simulink model "main_copy"  (R2023b)
settings: Solver=ode4  StartTime=0.0  StopTime=20  FixedStep=0.0001  RelTol=1e-3  AbsTol=1e-3  EnableMultiTasking=on
undefined symbols (not defined in the file or in its folder): X, Y, Z
libraries: sm_lib x84, nesl_utility x13, simulink_extras x3, ArmLibrary x2, gripper_v2_bottom x2, gripper_v2_top x2, lower_link_v2 x1, WorkSpaceLibrarry x1
settings Model: Creator=thiwa  LastModifiedBy=thiwa
settings SolverCC: AutoScaleAbsTol=off  AlgebraicLoopSolver=TrustRegion  MaxZcPerStep=1
settings DataIOCC: LimitDataPoints=on  MaxDataPoints=10000
settings OptimizationCC: ReuseModelBlockBuffer=off  LifeSpan=inf
settings DebuggingCC: UnconnectedInputMsg=warning  UnconnectedOutputMsg=warning  UnconnectedLineMsg=warning  AllowSymbolicDim=off  SubsystemReferenceDiagnosticForUnitTest=warning  SFUnexpectedBacktrackingDiag=warning  SFNoUnconditionalDefaultTransitionDiag=warning  SFExecutionAtInitializationDiag=none  ArithmeticOperatorsInVariantConditions=warning
settings ModelReferenceCC: EnableRefExpFcnMdlSchedulingChecks=on
settings SFSimCC: SimUseLocalCustomCode=off  CustomCodeUndefinedFunction=UseInterfaceOnly
settings RTWCC: RTWUseLocalCustomCode=off  DLArmComputeVersion=19.05
settings CodeAppCC: StateflowObjectComments=on
settings GRTTargetCC: TargetLangStandard=C89/C90 (ANSI)
settings ConfigComp: CovMetricSettings=dw  CovSaveCumulativeToWorkspaceVar=on  CovSaveSingleToWorkspaceVar=on  CovExternalEMLEnable=off  CovSFcnEnable=off
settings SimscapeCC: SimscapeLogType=all  SimscapeLogSimulationStatistics=on  SimscapeLogDataHistory=10000

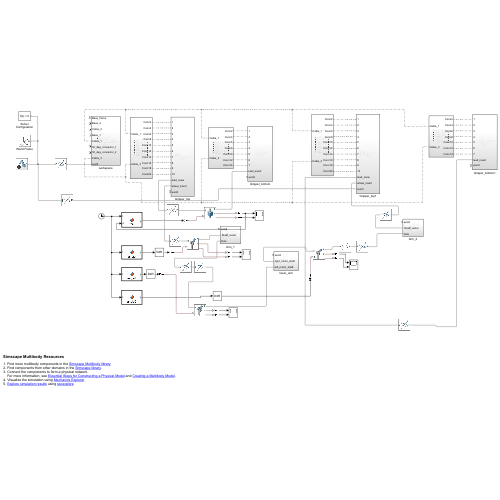
[thumbnail: Simulink's stored preview of the top-level diagram]
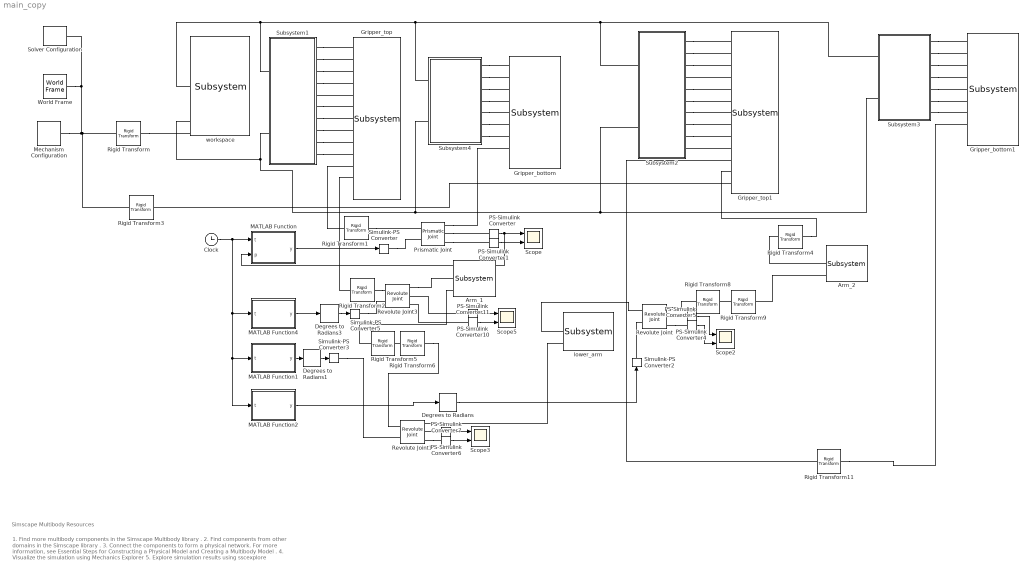
== system main_copy ==
  note: 1. Find more multibody components in the Simscape Multibody library .
      | 2. Find components from other domains in the Simscape library .
      | 3. Connect the components to form a physical network.
      | For more information, see Essential Steps for Constructing a Physical Model and Creating a Multibody Model .
      | 4. Visualize the simulation using Mechanics Explorer
      | 5. Explore simulation results using sscexplore
  note: Simscape Multibody Resources
  Arm_1 : ArmLibrary/Subsystem  SystemSampleTime=-1  VariantActivationTime=update diagram  AllowFlexibleInterface=on  Latency=0  AutoFrameSizeCalculation=off
  Arm_2 : ArmLibrary/Subsystem  SystemSampleTime=-1  VariantActivationTime=update diagram  AllowFlexibleInterface=on  Latency=0  AutoFrameSizeCalculation=off
  Clock : Clock
  Degrees to Radians : simulink_extras/Transformations/Degrees to Radians
  Degrees to Radians1 : simulink_extras/Transformations/Degrees to Radians
  Degrees to Radians3 : simulink_extras/Transformations/Degrees to Radians
  Gripper_bottom : gripper_v2_bottom/Subsystem  SystemSampleTime=-1  VariantActivationTime=update diagram  AllowFlexibleInterface=on  Latency=0  AutoFrameSizeCalculation=off
  Gripper_bottom1 : gripper_v2_bottom/Subsystem  SystemSampleTime=-1  VariantActivationTime=update diagram  AllowFlexibleInterface=on  Latency=0  AutoFrameSizeCalculation=off
  Gripper_top : gripper_v2_top/Subsystem  SystemSampleTime=-1  VariantActivationTime=update diagram  AllowFlexibleInterface=on  Latency=0  AutoFrameSizeCalculation=off
  Gripper_top1 : gripper_v2_top/Subsystem  SystemSampleTime=-1  VariantActivationTime=update diagram  AllowFlexibleInterface=on  Latency=0  AutoFrameSizeCalculation=off
  MATLAB Function : MATLAB Function  TreatAsAtomicUnit=on
  MATLAB Function1 : MATLAB Function  TreatAsAtomicUnit=on
  MATLAB Function2 : MATLAB Function  TreatAsAtomicUnit=on
  MATLAB Function4 : MATLAB Function  TreatAsAtomicUnit=on
  Mechanism Configuration : sm_lib/Utilities/Mechanism Configuration  UniformGravity=Constant  GravityVector=[0 0 -9.80665]  GravityVectorUnits=m/s^2  LinearizationDelta=0.001  JointModeTransitionNonlinearIterations=3
  PS-Simulink Converter{,1,4,6..7,10..11} (7 alike) : nesl_utility/PS-Simulink Converter  PhysicalDomain=network_engine_domain  SubClassName=ps_output  LeftPortType=input  RightPortType=output  PseudoPeriodic=off  Frequencies=[]  VectorFormat=inherit  Unit=inherit  AffineConversion=off
  PS-Simulink Converter5 : nesl_utility/PS-Simulink Converter  PhysicalDomain=network_engine_domain  SubClassName=ps_output  LeftPortType=input  RightPortType=output  PseudoPeriodic=off  Frequencies=[]  VectorFormat=inherit  Unit=N*m  AffineConversion=off
  Prismatic Joint : sm_lib/Joints/Prismatic Joint  JointMode=Normal  SenseConstraintForce=off  SenseConstraintForceX=off  SenseConstraintForceY=off  SenseConstraintForceZ=off  SenseConstraintTorque=off  SenseConstraintTorqueX=off  SenseConstraintTorqueY=off  SenseConstraintTorqueZ=off  SenseTotalForce=off  SenseTotalForceX=off  SenseTotalForceY=off  SenseTotalForceZ=off  SenseTotalTorque=off  SenseTotalTorqueX=off  SenseTotalTorqueY=off  SenseTotalTorqueZ=off  CompositeWrenchDir=FollowerOnBase  CompositeWrenchFrame=BaseFrame  EquilibriumPosition=0  EquilibriumPositionUnits=m  SpringStiffness=0  SpringStiffnessUnits=N/m  DampingCoefficient=10  DampingCoefficientUnits=N/(m/s)  TorqueActuationMode=InputTorque  MotionActuationMode=ComputedMotion  SensePosition=on  SenseVelocity=off  SenseAcceleration=off  SenseTorqueForce=on  SenseLowerLimitTorqueForce=off  SenseUpperLimitTorqueForce=off  LowerLimitSpecify=off  LowerLimitBound=-1  LowerLimitBoundUnits=m  LowerLimitStiffness=1e6  LowerLimitStiffnessUnits=N/m  LowerLimitDamping=1e3  LowerLimitDampingUnits=N/(m/s)  LowerLimitTransitionRegionWidth=1e-4  LowerLimitTransitionRegionWidthUnits=m  UpperLimitSpecify=off  UpperLimitBound=1  UpperLimitBoundUnits=m  UpperLimitStiffness=1e6  UpperLimitStiffnessUnits=N/m  UpperLimitDamping=1e3  UpperLimitDampingUnits=N/(m/s)  UpperLimitTransitionRegionWidth=1e-4  UpperLimitTransitionRegionWidthUnits=m  PositionTargetSpecify=on  PositionTargetPriority=High  PositionTargetValue=-50  PositionTargetValueUnits=mm  VelocityTargetSpecify=off  VelocityTargetPriority=High  VelocityTargetValue=0  VelocityTargetValueUnits=m/s
  Revolute Joint : sm_lib/Joints/Revolute Joint  JointMode=Normal  SenseConstraintForce=off  SenseConstraintForceX=off  SenseConstraintForceY=off  SenseConstraintForceZ=off  SenseConstraintTorque=off  SenseConstraintTorqueX=off  SenseConstraintTorqueY=off  SenseConstraintTorqueZ=off  SenseTotalForce=off  SenseTotalForceX=off  SenseTotalForceY=off  SenseTotalForceZ=off  SenseTotalTorque=off  SenseTotalTorqueX=off  SenseTotalTorqueY=off  SenseTotalTorqueZ=off  CompositeWrenchDir=FollowerOnBase  CompositeWrenchFrame=BaseFrame  EquilibriumPosition=0  EquilibriumPositionUnits=deg  SpringStiffness=0  SpringStiffnessUnits=N*m/deg  DampingCoefficient=1  DampingCoefficientUnits=N*m/(deg/s)  TorqueActuationMode=ComputedTorque  MotionActuationMode=InputMotion  SensePosition=on  SenseVelocity=off  SenseAcceleration=off  SenseTorqueForce=on  SenseLowerLimitTorqueForce=off  SenseUpperLimitTorqueForce=off  LowerLimitSpecify=off  LowerLimitBound=-90  LowerLimitBoundUnits=deg  LowerLimitStiffness=1e4  LowerLimitStiffnessUnits=N*m/deg  LowerLimitDamping=10  LowerLimitDampingUnits=N*m/(deg/s)  LowerLimitTransitionRegionWidth=0.1  LowerLimitTransitionRegionWidthUnits=deg  UpperLimitSpecify=off  UpperLimitBound=90  UpperLimitBoundUnits=deg  UpperLimitStiffness=1e4  UpperLimitStiffnessUnits=N*m/deg  UpperLimitDamping=10  UpperLimitDampingUnits=N*m/(deg/s)  UpperLimitTransitionRegionWidth=0.1  UpperLimitTransitionRegionWidthUnits=deg  PositionTargetSpecify=on  PositionTargetPriority=High  PositionTargetValue=0  PositionTargetValueUnits=deg  VelocityTargetSpecify=off  VelocityTargetPriority=High  VelocityTargetValue=0  VelocityTargetValueUnits=deg/s
  Revolute Joint1 : sm_lib/Joints/Revolute Joint  JointMode=Normal  SenseConstraintForce=off  SenseConstraintForceX=off  SenseConstraintForceY=off  SenseConstraintForceZ=off  SenseConstraintTorque=off  SenseConstraintTorqueX=off  SenseConstraintTorqueY=off  SenseConstraintTorqueZ=off  SenseTotalForce=off  SenseTotalForceX=off  SenseTotalForceY=off  SenseTotalForceZ=off  SenseTotalTorque=off  SenseTotalTorqueX=off  SenseTotalTorqueY=off  SenseTotalTorqueZ=off  CompositeWrenchDir=FollowerOnBase  CompositeWrenchFrame=BaseFrame  EquilibriumPosition=0  EquilibriumPositionUnits=deg  SpringStiffness=0  SpringStiffnessUnits=N*m/deg  DampingCoefficient=1  DampingCoefficientUnits=N*m/(deg/s)  TorqueActuationMode=ComputedTorque  MotionActuationMode=InputMotion  SensePosition=on  SenseVelocity=off  SenseAcceleration=off  SenseTorqueForce=on  SenseLowerLimitTorqueForce=off  SenseUpperLimitTorqueForce=off  LowerLimitSpecify=off  LowerLimitBound=-90  LowerLimitBoundUnits=deg  LowerLimitStiffness=1e4  LowerLimitStiffnessUnits=N*m/deg  LowerLimitDamping=10  LowerLimitDampingUnits=N*m/(deg/s)  LowerLimitTransitionRegionWidth=0.1  LowerLimitTransitionRegionWidthUnits=deg  UpperLimitSpecify=off  UpperLimitBound=90  UpperLimitBoundUnits=deg  UpperLimitStiffness=1e4  UpperLimitStiffnessUnits=N*m/deg  UpperLimitDamping=10  UpperLimitDampingUnits=N*m/(deg/s)  UpperLimitTransitionRegionWidth=0.1  UpperLimitTransitionRegionWidthUnits=deg  PositionTargetSpecify=on  PositionTargetPriority=High  PositionTargetValue=-90  PositionTargetValueUnits=deg  VelocityTargetSpecify=off  VelocityTargetPriority=High  VelocityTargetValue=0  VelocityTargetValueUnits=deg/s
  Revolute Joint3 : sm_lib/Joints/Revolute Joint  JointMode=Normal  SenseConstraintForce=off  SenseConstraintForceX=off  SenseConstraintForceY=off  SenseConstraintForceZ=off  SenseConstraintTorque=off  SenseConstraintTorqueX=off  SenseConstraintTorqueY=off  SenseConstraintTorqueZ=off  SenseTotalForce=off  SenseTotalForceX=off  SenseTotalForceY=off  SenseTotalForceZ=off  SenseTotalTorque=off  SenseTotalTorqueX=off  SenseTotalTorqueY=off  SenseTotalTorqueZ=off  CompositeWrenchDir=FollowerOnBase  CompositeWrenchFrame=BaseFrame  EquilibriumPosition=0  EquilibriumPositionUnits=deg  SpringStiffness=0  SpringStiffnessUnits=N*m/deg  DampingCoefficient=1  DampingCoefficientUnits=N*m/(deg/s)  TorqueActuationMode=ComputedTorque  MotionActuationMode=InputMotion  SensePosition=on  SenseVelocity=off  SenseAcceleration=off  SenseTorqueForce=on  SenseLowerLimitTorqueForce=off  SenseUpperLimitTorqueForce=off  LowerLimitSpecify=off  LowerLimitBound=-90  LowerLimitBoundUnits=deg  LowerLimitStiffness=1e4  LowerLimitStiffnessUnits=N*m/deg  LowerLimitDamping=10  LowerLimitDampingUnits=N*m/(deg/s)  LowerLimitTransitionRegionWidth=0.1  LowerLimitTransitionRegionWidthUnits=deg  UpperLimitSpecify=off  UpperLimitBound=90  UpperLimitBoundUnits=deg  UpperLimitStiffness=1e4  UpperLimitStiffnessUnits=N*m/deg  UpperLimitDamping=10  UpperLimitDampingUnits=N*m/(deg/s)  UpperLimitTransitionRegionWidth=0.1  UpperLimitTransitionRegionWidthUnits=deg  PositionTargetSpecify=on  PositionTargetPriority=High  PositionTargetValue=-90-25.5  PositionTargetValueUnits=deg  VelocityTargetSpecify=off  VelocityTargetPriority=High  VelocityTargetValue=0  VelocityTargetValueUnits=deg/s
  Rigid Transform : sm_lib/Frames and Transforms/Rigid Transform  TranslationMethod=None  TranslationStandardOffset=0  TranslationStandardOffsetUnits=m  TranslationStandardAxis=+Z  TranslationCartesianOffset=[0 0 0]  TranslationCartesianOffsetUnits=m  TranslationROffset=0  TranslationROffsetUnits=m  TranslationZOffset=0  TranslationZOffsetUnits=m  TranslationThetaOffset=0  TranslationThetaOffsetUnits=deg  RotationMethod=StandardAxis  RotationAngleUnits=deg  RotationStandardAxis=+Y  RotationAngle=180  RotationArbitraryAxis=[0 0 1]  FollAlignAxisA=+X  BaseAlignAxisA=+Y  FollAlignAxisB=+Y  BaseAlignAxisB=+Z  RotationSequenceAxes=FollowerAxes  RotationSequence=XYX  RotationSequenceAngles=[0 0 0]  RotationSequenceAnglesUnits=deg  RotationMatrix=[1 0 0; 0 1 0; 0 0 1]  Quaternion=[1 0 0 0]
  Rigid Transform1 : sm_lib/Frames and Transforms/Rigid Transform  TranslationMethod=None  TranslationStandardOffset=0  TranslationStandardOffsetUnits=m  TranslationStandardAxis=+Z  TranslationCartesianOffset=[0 0 0]  TranslationCartesianOffsetUnits=m  TranslationROffset=0  TranslationROffsetUnits=m  TranslationZOffset=0  TranslationZOffsetUnits=m  TranslationThetaOffset=0  TranslationThetaOffsetUnits=deg  RotationMethod=StandardAxis  RotationAngleUnits=deg  RotationStandardAxis=+Y  RotationAngle=180  RotationArbitraryAxis=[0 0 1]  FollAlignAxisA=+X  BaseAlignAxisA=+Y  FollAlignAxisB=+Y  BaseAlignAxisB=+Z  RotationSequenceAxes=FollowerAxes  RotationSequence=XYX  RotationSequenceAngles=[0 0 0]  RotationSequenceAnglesUnits=deg  RotationMatrix=[1 0 0; 0 1 0; 0 0 1]  Quaternion=[1 0 0 0]
  Rigid Transform11 : sm_lib/Frames and Transforms/Rigid Transform  TranslationMethod=StandardAxis  TranslationStandardOffset=50  TranslationStandardOffsetUnits=mm  TranslationStandardAxis=+Z  TranslationCartesianOffset=[0 0 0]  TranslationCartesianOffsetUnits=m  TranslationROffset=0  TranslationROffsetUnits=m  TranslationZOffset=0  TranslationZOffsetUnits=m  TranslationThetaOffset=0  TranslationThetaOffsetUnits=deg  RotationMethod=StandardAxis  RotationAngleUnits=deg  RotationStandardAxis=+Y  RotationAngle=180  RotationArbitraryAxis=[0 0 1]  FollAlignAxisA=+X  BaseAlignAxisA=+Y  FollAlignAxisB=+Y  BaseAlignAxisB=+Z  RotationSequenceAxes=FollowerAxes  RotationSequence=XYX  RotationSequenceAngles=[0 0 0]  RotationSequenceAnglesUnits=deg  RotationMatrix=[1 0 0; 0 1 0; 0 0 1]  Quaternion=[1 0 0 0]
  Rigid Transform2 : sm_lib/Frames and Transforms/Rigid Transform  TranslationMethod=StandardAxis  TranslationStandardOffset=12  TranslationStandardOffsetUnits=mm  TranslationStandardAxis=-Z  TranslationCartesianOffset=[0 0 0]  TranslationCartesianOffsetUnits=m  TranslationROffset=0  TranslationROffsetUnits=m  TranslationZOffset=0  TranslationZOffsetUnits=m  TranslationThetaOffset=0  TranslationThetaOffsetUnits=deg  RotationMethod=None  RotationAngleUnits=deg  RotationStandardAxis=+Z  RotationAngle=0.0  RotationArbitraryAxis=[0 0 1]  FollAlignAxisA=+X  BaseAlignAxisA=+Y  FollAlignAxisB=+Y  BaseAlignAxisB=+Z  RotationSequenceAxes=FollowerAxes  RotationSequence=XYX  RotationSequenceAngles=[0 0 0]  RotationSequenceAnglesUnits=deg  RotationMatrix=[1 0 0; 0 1 0; 0 0 1]  Quaternion=[1 0 0 0]
  Rigid Transform3 : sm_lib/Frames and Transforms/Rigid Transform  TranslationMethod=None  TranslationStandardOffset=0  TranslationStandardOffsetUnits=m  TranslationStandardAxis=+Z  TranslationCartesianOffset=[0 0 0]  TranslationCartesianOffsetUnits=m  TranslationROffset=0  TranslationROffsetUnits=m  TranslationZOffset=0  TranslationZOffsetUnits=m  TranslationThetaOffset=0  TranslationThetaOffsetUnits=deg  RotationMethod=StandardAxis  RotationAngleUnits=deg  RotationStandardAxis=+Y  RotationAngle=180  RotationArbitraryAxis=[0 0 1]  FollAlignAxisA=+X  BaseAlignAxisA=+Y  FollAlignAxisB=+Y  BaseAlignAxisB=+Z  RotationSequenceAxes=FollowerAxes  RotationSequence=XYX  RotationSequenceAngles=[0 0 0]  RotationSequenceAnglesUnits=deg  RotationMatrix=[1 0 0; 0 1 0; 0 0 1]  Quaternion=[1 0 0 0]
  Rigid Transform4 : sm_lib/Frames and Transforms/Rigid Transform  TranslationMethod=None  TranslationStandardOffset=0  TranslationStandardOffsetUnits=m  TranslationStandardAxis=+Z  TranslationCartesianOffset=[0 0 0]  TranslationCartesianOffsetUnits=m  TranslationROffset=0  TranslationROffsetUnits=m  TranslationZOffset=0  TranslationZOffsetUnits=m  TranslationThetaOffset=0  TranslationThetaOffsetUnits=deg  RotationMethod=StandardAxis  RotationAngleUnits=deg  RotationStandardAxis=+Z  RotationAngle=25.5+90  RotationArbitraryAxis=[0 0 1]  FollAlignAxisA=+X  BaseAlignAxisA=+Y  FollAlignAxisB=+Y  BaseAlignAxisB=+Z  RotationSequenceAxes=FollowerAxes  RotationSequence=XYX  RotationSequenceAngles=[0 0 0]  RotationSequenceAnglesUnits=deg  RotationMatrix=[1 0 0; 0 1 0; 0 0 1]  Quaternion=[1 0 0 0]
  Rigid Transform5 : sm_lib/Frames and Transforms/Rigid Transform  TranslationMethod=None  TranslationStandardOffset=0  TranslationStandardOffsetUnits=m  TranslationStandardAxis=+Z  TranslationCartesianOffset=[0 0 0]  TranslationCartesianOffsetUnits=m  TranslationROffset=0  TranslationROffsetUnits=m  TranslationZOffset=0  TranslationZOffsetUnits=m  TranslationThetaOffset=0  TranslationThetaOffsetUnits=deg  RotationMethod=StandardAxis  RotationAngleUnits=deg  RotationStandardAxis=+Y  RotationAngle=90  RotationArbitraryAxis=[0 0 1]  FollAlignAxisA=+X  BaseAlignAxisA=+Y  FollAlignAxisB=+Y  BaseAlignAxisB=+Z  RotationSequenceAxes=FollowerAxes  RotationSequence=XYX  RotationSequenceAngles=[0 0 0]  RotationSequenceAnglesUnits=deg  RotationMatrix=[1 0 0; 0 1 0; 0 0 1]  Quaternion=[1 0 0 0]
  Rigid Transform6 : sm_lib/Frames and Transforms/Rigid Transform  TranslationMethod=None  TranslationStandardOffset=0  TranslationStandardOffsetUnits=m  TranslationStandardAxis=+Z  TranslationCartesianOffset=[0 0 0]  TranslationCartesianOffsetUnits=m  TranslationROffset=0  TranslationROffsetUnits=m  TranslationZOffset=0  TranslationZOffsetUnits=m  TranslationThetaOffset=0  TranslationThetaOffsetUnits=deg  RotationMethod=StandardAxis  RotationAngleUnits=deg  RotationStandardAxis=+X  RotationAngle=180  RotationArbitraryAxis=[0 0 1]  FollAlignAxisA=+X  BaseAlignAxisA=+Y  FollAlignAxisB=+Y  BaseAlignAxisB=+Z  RotationSequenceAxes=FollowerAxes  RotationSequence=XYX  RotationSequenceAngles=[0 0 0]  RotationSequenceAnglesUnits=deg  RotationMatrix=[1 0 0; 0 1 0; 0 0 1]  Quaternion=[1 0 0 0]
  Rigid Transform8 : sm_lib/Frames and Transforms/Rigid Transform  TranslationMethod=None  TranslationStandardOffset=0  TranslationStandardOffsetUnits=m  TranslationStandardAxis=+Z  TranslationCartesianOffset=[0 0 0]  TranslationCartesianOffsetUnits=m  TranslationROffset=0  TranslationROffsetUnits=m  TranslationZOffset=0  TranslationZOffsetUnits=m  TranslationThetaOffset=0  TranslationThetaOffsetUnits=deg  RotationMethod=StandardAxis  RotationAngleUnits=deg  RotationStandardAxis=+Y  RotationAngle=90  RotationArbitraryAxis=[0 0 1]  FollAlignAxisA=+X  BaseAlignAxisA=+Y  FollAlignAxisB=+Y  BaseAlignAxisB=+Z  RotationSequenceAxes=FollowerAxes  RotationSequence=XYX  RotationSequenceAngles=[0 0 0]  RotationSequenceAnglesUnits=deg  RotationMatrix=[1 0 0; 0 1 0; 0 0 1]  Quaternion=[1 0 0 0]
  Rigid Transform9 : sm_lib/Frames and Transforms/Rigid Transform  TranslationMethod=None  TranslationStandardOffset=0  TranslationStandardOffsetUnits=m  TranslationStandardAxis=+Z  TranslationCartesianOffset=[0 0 0]  TranslationCartesianOffsetUnits=m  TranslationROffset=0  TranslationROffsetUnits=m  TranslationZOffset=0  TranslationZOffsetUnits=m  TranslationThetaOffset=0  TranslationThetaOffsetUnits=deg  RotationMethod=StandardAxis  RotationAngleUnits=deg  RotationStandardAxis=+X  RotationAngle=90  RotationArbitraryAxis=[0 0 1]  FollAlignAxisA=+X  BaseAlignAxisA=+Y  FollAlignAxisB=+Y  BaseAlignAxisB=+Z  RotationSequenceAxes=FollowerAxes  RotationSequence=XYX  RotationSequenceAngles=[0 0 0]  RotationSequenceAnglesUnits=deg  RotationMatrix=[1 0 0; 0 1 0; 0 0 1]  Quaternion=[1 0 0 0]
  Scope{,2..3,5} (4 alike) : Scope  NumInputPorts=2
  Simulink-PS Converter : nesl_utility/Simulink-PS Converter  PhysicalDomain=network_engine_domain  SubClassName=ps_input  LeftPortType=input  RightPortType=output  PseudoPeriodic=off  Frequencies=[]  NoiseDistribution=none  NoiseParameters=[]  Unit=1  AffineConversion=off  FilteringAndDerivatives=provide  SimscapeFilterOrder=1  InputFilterTimeConstant=0.001  UdotUserProvided=0
  Simulink-PS Converter2 : nesl_utility/Simulink-PS Converter  PhysicalDomain=network_engine_domain  SubClassName=ps_input  LeftPortType=input  RightPortType=output  PseudoPeriodic=off  Frequencies=[]  NoiseDistribution=none  NoiseParameters=[]  Unit=1  AffineConversion=off  FilteringAndDerivatives=filter  SimscapeFilterOrder=2  InputFilterTimeConstant=0.001  UdotUserProvided=0
  Simulink-PS Converter3 : nesl_utility/Simulink-PS Converter  PhysicalDomain=network_engine_domain  SubClassName=ps_input  LeftPortType=input  RightPortType=output  PseudoPeriodic=off  Frequencies=[]  NoiseDistribution=none  NoiseParameters=[]  Unit=1  AffineConversion=off  FilteringAndDerivatives=filter  SimscapeFilterOrder=2  InputFilterTimeConstant=0.001  UdotUserProvided=0
  Simulink-PS Converter5 : nesl_utility/Simulink-PS Converter  PhysicalDomain=network_engine_domain  SubClassName=ps_input  LeftPortType=input  RightPortType=output  PseudoPeriodic=off  Frequencies=[]  NoiseDistribution=none  NoiseParameters=[]  Unit=1  AffineConversion=off  FilteringAndDerivatives=filter  SimscapeFilterOrder=2  InputFilterTimeConstant=0.001  UdotUserProvided=0
  Solver Configuration : nesl_utility/Solver Configuration  PhysicalDomain=network_engine_domain  SubClassName=solver  LeftPortType=input  RightPortType=generic  Tones=[]  Harmonics=[]  SimulateNoise=off  Profile=off  UseLocalSampling=off  EnableSwitchedLinearOptims=on  FrequencyDomain=off  UseCCode=off  RelTol=0.001  AbsTol=1e-06  MinStep=1e-09  ToWorkspace=off  RevertToSquareIcSolve=off  NumHomotopyIterations=100  PhasorMode=off  PhasorModeNumHarmonics=1  ConsistencySolver=NEWTON_XTOL_AFTER_FTOL  IndexReductionMethod=DerivativeReplacement  DoDC=off  ResidualTolerance=1e-09  ConsistencyTolSource=GLOBAL  ConsistencyAbsTol=0.001  ConsistencyRelTol=0.001  ConsistencyTolFactor=0.001  UseLocalSolver=off  LocalSolverChoice=NE_BACKWARD_EULER_ADVANCER  ResolveIndetEquations=on  FunctionEvalNumThread=1  LocalSolverSampleTime=0.001  DoFixedCost=off  MaxNonlinIter=3  MaxModeIter=2  ComputeImpulses=off  ImpulseIterations=2  LinearAlgebra=Sparse  LinearAlgebraNumThread=0  EquationFormulation=NE_TIME_EF  DelaysMemoryBudget=1024  AutomaticFiltering=on  FilteringTimeConstant=0.001  PartitionStorageMethod=AS_NEEDED  PartitionMemoryBudget=1024  PartitionMethod=FAST  MultibodyUseLocalSolver=off  MultibodyLocalSolverChoice=ODE1  MultibodyLocalSolverSampleTime=0.001
  Subsystem1 : Subsystem
  Subsystem2 : Subsystem
  Subsystem3 : Subsystem
  Subsystem4 : Subsystem
  World Frame : sm_lib/Frames and Transforms/World Frame
  lower_arm : lower_link_v2/Subsystem  SystemSampleTime=-1  VariantActivationTime=update diagram  AllowFlexibleInterface=on  Latency=0  AutoFrameSizeCalculation=off
  workspace : WorkSpaceLibrarry/Subsystem  SystemSampleTime=-1  VariantActivationTime=update diagram  AllowFlexibleInterface=on  Latency=0  AutoFrameSizeCalculation=off
      link override Cable_3_RIGID/Solid: ExtGeomFileName=C:\Thiwanka\Assignments\Cable_Inspection_Robot\Design\Simscapetest_3\Workspace_Frame\Cable_100_long_sldprt.STEP
  wires:
  PS-Simulink Converter1/1 -> Scope/2
  PS-Simulink Converter/1 -> MATLAB Function/2(p), Scope/1
  MATLAB Function/1(y) -> Simulink-PS Converter/1
  Clock/1 -> MATLAB Function/1(t), MATLAB Function4/1(t), MATLAB Function1/1(t), MATLAB Function2/1(t)
  PS-Simulink Converter7/1 -> Scope3/2
  PS-Simulink Converter6/1 -> Scope3/1
  Degrees to Radians1/1 -> Simulink-PS Converter3/1
  MATLAB Function1/1(y) -> Degrees to Radians1/1
  PS-Simulink Converter10/1 -> Scope5/1
  PS-Simulink Converter11/1 -> Scope5/2
  Degrees to Radians3/1 -> Simulink-PS Converter5/1
  MATLAB Function4/1(y) -> Degrees to Radians3/1
  MATLAB Function2/1(y) -> Degrees to Radians/1
  Degrees to Radians/1 -> Simulink-PS Converter2/1
  PS-Simulink Converter4/1 -> Scope2/1
  PS-Simulink Converter5/1 -> Scope2/2
  connections:
  Rigid Transform/RConn1 -- workspace/LConn9
  Prismatic Joint/RConn1 -- Gripper_bottom/LConn8
  Rigid Transform2/LConn1 -- Gripper_top/LConn12
  Rigid Transform6/LConn1 -- Rigid Transform5/RConn1
  Rigid Transform9/LConn1 -- Rigid Transform8/RConn1
  Rigid Transform11/LConn1 -- Gripper_top1/LConn11
  Rigid Transform1/RConn1 -- Prismatic Joint/LConn1
  Prismatic Joint/RConn2 -- PS-Simulink Converter/LConn1
  Prismatic Joint/RConn3 -- PS-Simulink Converter1/LConn1
  Simulink-PS Converter/RConn1 -- Prismatic Joint/LConn2
  Rigid Transform11/RConn1 -- Gripper_bottom1/LConn8
  World Frame/RConn1 -- Rigid Transform3/LConn1 -- Rigid Transform/LConn1 -- Mechanism Configuration/RConn1 -- Solver Configuration/RConn1
  lower_arm/LConn2 -- Revolute Joint/LConn1
  Revolute Joint/RConn1 -- Rigid Transform8/LConn1
  Revolute Joint1/RConn2 -- PS-Simulink Converter6/LConn1
  Revolute Joint1/RConn3 -- PS-Simulink Converter7/LConn1
  Simulink-PS Converter3/RConn1 -- Revolute Joint1/LConn2
  Rigid Transform5/LConn1 -- Arm_1/LConn3
  Rigid Transform6/RConn1 -- Revolute Joint1/LConn1
  Revolute Joint1/RConn1 -- lower_arm/LConn3
  Subsystem4/RConn1 -- Gripper_bottom/LConn1
  Subsystem4/RConn2 -- Gripper_bottom/LConn2
  Subsystem4/RConn3 -- Gripper_bottom/LConn3
  Subsystem4/RConn4 -- Gripper_bottom/LConn4
  Subsystem4/RConn5 -- Gripper_bottom/LConn5
  Subsystem4/RConn6 -- Gripper_bottom/LConn6
  Subsystem4/RConn7 -- Gripper_bottom/LConn7
  Subsystem1/RConn10 -- Gripper_top/LConn10
  Subsystem1/RConn9 -- Gripper_top/LConn9
  Subsystem1/RConn8 -- Gripper_top/LConn8
  Subsystem1/RConn7 -- Gripper_top/LConn7
  Subsystem1/RConn6 -- Gripper_top/LConn6
  Gripper_top/LConn5 -- Subsystem1/RConn5
  Subsystem1/RConn4 -- Gripper_top/LConn4
  Subsystem1/RConn3 -- Gripper_top/LConn3
  Subsystem1/RConn2 -- Gripper_top/LConn2
  Subsystem1/RConn1 -- Gripper_top/LConn1
  workspace/LConn5 -- Subsystem3/LConn1 -- Subsystem2/LConn1 -- Subsystem4/LConn1 -- Subsystem1/LConn1
  Subsystem1/LConn2 -- Subsystem2/LConn2 -- Subsystem3/LConn2 -- Subsystem4/LConn2 -- workspace/LConn8
  Subsystem2/RConn1 -- Gripper_top1/LConn1
  Subsystem2/RConn2 -- Gripper_top1/LConn2
  Subsystem2/RConn3 -- Gripper_top1/LConn3
  Gripper_top1/LConn4 -- Subsystem2/RConn4
  Subsystem2/RConn5 -- Gripper_top1/LConn5
  Subsystem2/RConn6 -- Gripper_top1/LConn6
  Subsystem2/RConn7 -- Gripper_top1/LConn7
  Subsystem2/RConn8 -- Gripper_top1/LConn8
  Subsystem2/RConn9 -- Gripper_top1/LConn9
  Gripper_top1/LConn10 -- Subsystem2/RConn10
  Subsystem3/RConn1 -- Gripper_bottom1/LConn1
  Subsystem3/RConn2 -- Gripper_bottom1/LConn2
  Subsystem3/RConn3 -- Gripper_bottom1/LConn3
  Subsystem3/RConn4 -- Gripper_bottom1/LConn4
  Subsystem3/RConn5 -- Gripper_bottom1/LConn5
  Subsystem3/RConn6 -- Gripper_bottom1/LConn6
  Subsystem3/RConn7 -- Gripper_bottom1/LConn7
  Rigid Transform2/RConn1 -- Revolute Joint3/LConn1
  Revolute Joint3/RConn1 -- Arm_1/LConn2
  PS-Simulink Converter10/LConn1 -- Revolute Joint3/RConn2
  PS-Simulink Converter11/LConn1 -- Revolute Joint3/RConn3
  Simulink-PS Converter5/RConn1 -- Revolute Joint3/LConn2
  Arm_2/LConn3 -- Rigid Transform9/RConn1
  Simulink-PS Converter2/RConn1 -- Revolute Joint/LConn2
  Revolute Joint/RConn2 -- PS-Simulink Converter4/LConn1
  Revolute Joint/RConn3 -- PS-Simulink Converter5/LConn1
  Gripper_top/LConn11 -- Rigid Transform1/LConn1
  Gripper_top1/LConn13 -- Rigid Transform3/RConn1
  Arm_2/LConn2 -- Rigid Transform4/LConn1
  Rigid Transform4/RConn1 -- Gripper_top1/LConn12

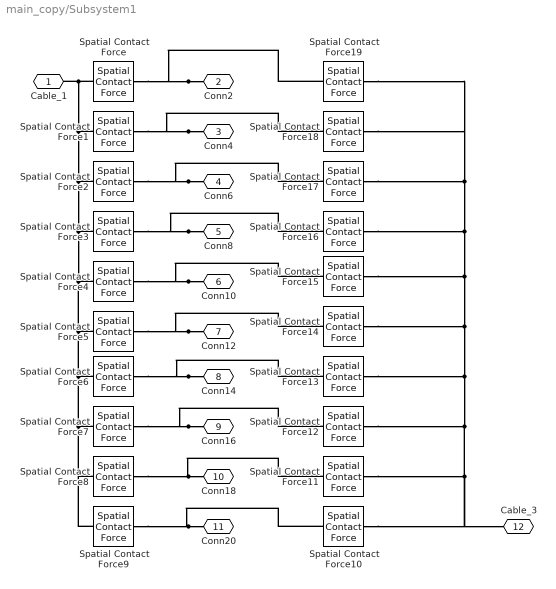
== system main_copy/Subsystem1 ==
  Spatial Contact Force{,1..19} (20 alike) : sm_lib/Forces and Torques/Spatial Contact Force  SenseContactBaseRotation=off  SenseContactBaseTranslation=off  CoefficientOfDynamicFriction=0.3  CoefficientOfStaticFriction=0.5  NormalDamping=1e3  NormalDampingUnits=N/(m/s)  SenseContactSignal=off  NormalStiffness=1e6  NormalStiffnessUnits=N/m  FrictionalCriticalVelocity=1e-3  FrictionalCriticalVelocityUnits=m/s  ZeroCrossDetectContactStartAndEnd=off  SenseContactFollowerRotation=off  SenseContactFollowerTranslation=off  FrictionType=SmoothStickSlip  SenseFrictionalForceMagnitude=off  SenseNormalForceMagnitude=off  NormalForceType=SmoothSpringDamper  SenseNormalVelocity=off  SensePenetrationDepth=off  SenseSeparationDistance=off  SenseTangentialVelocity=off  NormalTransitionRegionWidth=1e-4  NormalTransitionRegionWidthUnits=m
  Cable_1 : PMIOPort  Side=Left
  Conn2 : PMIOPort  Port=2  Side=Right
  Conn4 : PMIOPort  Port=3  Side=Right
  Conn6 : PMIOPort  Port=4  Side=Right
  Conn8 : PMIOPort  Port=5  Side=Right
  Conn10 : PMIOPort  Port=6  Side=Right
  Conn12 : PMIOPort  Port=7  Side=Right
  Conn14 : PMIOPort  Port=8  Side=Right
  Conn16 : PMIOPort  Port=9  Side=Right
  Conn18 : PMIOPort  Port=10  Side=Right
  Conn20 : PMIOPort  Port=11  Side=Right
  Cable_3 : PMIOPort  Port=12  Side=Left
  connections:
  Spatial Contact Force15/LConn1 -- Spatial Contact Force14/LConn1 -- Spatial Contact Force13/LConn1 -- Spatial Contact Force11/LConn1 -- Cable_3/RConn1 -- Spatial Contact Force10/LConn1 -- Spatial Contact Force12/LConn1 -- Spatial Contact Force17/LConn1 -- Spatial Contact Force18/LConn1 -- Spatial Contact Force19/LConn1 -- Spatial Contact Force16/LConn1
  Conn20/RConn1 -- Spatial Contact Force10/RConn1 -- Spatial Contact Force9/RConn1
  Conn16/RConn1 -- Spatial Contact Force12/RConn1 -- Spatial Contact Force7/RConn1
  Conn18/RConn1 -- Spatial Contact Force11/RConn1 -- Spatial Contact Force8/RConn1
  Conn14/RConn1 -- Spatial Contact Force13/RConn1 -- Spatial Contact Force6/RConn1
  Conn8/RConn1 -- Spatial Contact Force16/RConn1 -- Spatial Contact Force3/RConn1
  Conn10/RConn1 -- Spatial Contact Force15/RConn1 -- Spatial Contact Force4/RConn1
  Conn12/RConn1 -- Spatial Contact Force14/RConn1 -- Spatial Contact Force5/RConn1
  Conn6/RConn1 -- Spatial Contact Force17/RConn1 -- Spatial Contact Force2/RConn1
  Cable_1/RConn1 -- Spatial Contact Force1/LConn1 -- Spatial Contact Force2/LConn1 -- Spatial Contact Force3/LConn1 -- Spatial Contact Force4/LConn1 -- Spatial Contact Force5/LConn1 -- Spatial Contact Force6/LConn1 -- Spatial Contact Force7/LConn1 -- Spatial Contact Force8/LConn1 -- Spatial Contact Force9/LConn1 -- Spatial Contact Force/LConn1
  Conn4/RConn1 -- Spatial Contact Force18/RConn1 -- Spatial Contact Force1/RConn1
  Conn2/RConn1 -- Spatial Contact Force19/RConn1 -- Spatial Contact Force/RConn1

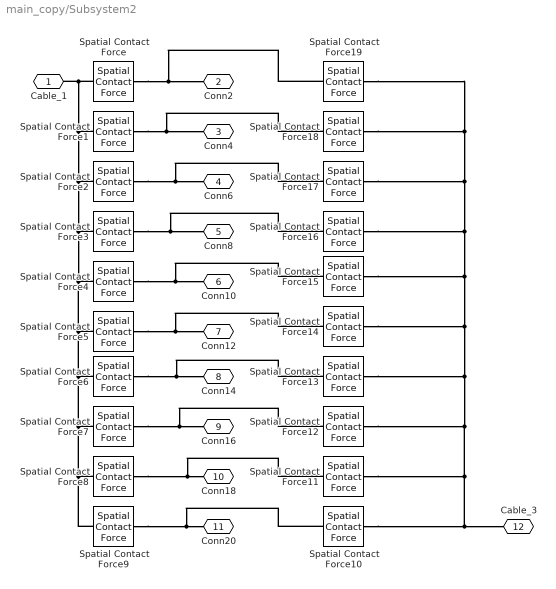
== system main_copy/Subsystem2 ==
  Spatial Contact Force{,1..19} (20 alike) : sm_lib/Forces and Torques/Spatial Contact Force  SenseContactBaseRotation=off  SenseContactBaseTranslation=off  CoefficientOfDynamicFriction=0.3  CoefficientOfStaticFriction=0.5  NormalDamping=1e3  NormalDampingUnits=N/(m/s)  SenseContactSignal=off  NormalStiffness=1e6  NormalStiffnessUnits=N/m  FrictionalCriticalVelocity=1e-3  FrictionalCriticalVelocityUnits=m/s  ZeroCrossDetectContactStartAndEnd=off  SenseContactFollowerRotation=off  SenseContactFollowerTranslation=off  FrictionType=SmoothStickSlip  SenseFrictionalForceMagnitude=off  SenseNormalForceMagnitude=off  NormalForceType=SmoothSpringDamper  SenseNormalVelocity=off  SensePenetrationDepth=off  SenseSeparationDistance=off  SenseTangentialVelocity=off  NormalTransitionRegionWidth=1e-4  NormalTransitionRegionWidthUnits=m
  Cable_1 : PMIOPort  Side=Left
  Conn2 : PMIOPort  Port=2  Side=Right
  Conn4 : PMIOPort  Port=3  Side=Right
  Conn6 : PMIOPort  Port=4  Side=Right
  Conn8 : PMIOPort  Port=5  Side=Right
  Conn10 : PMIOPort  Port=6  Side=Right
  Conn12 : PMIOPort  Port=7  Side=Right
  Conn14 : PMIOPort  Port=8  Side=Right
  Conn16 : PMIOPort  Port=9  Side=Right
  Conn18 : PMIOPort  Port=10  Side=Right
  Conn20 : PMIOPort  Port=11  Side=Right
  Cable_3 : PMIOPort  Port=12  Side=Left
  connections:
  Spatial Contact Force/RConn1 -- Spatial Contact Force19/RConn1 -- Conn2/RConn1
  Spatial Contact Force1/RConn1 -- Spatial Contact Force18/RConn1 -- Conn4/RConn1
  Spatial Contact Force/LConn1 -- Spatial Contact Force9/LConn1 -- Spatial Contact Force8/LConn1 -- Spatial Contact Force7/LConn1 -- Spatial Contact Force6/LConn1 -- Spatial Contact Force5/LConn1 -- Spatial Contact Force4/LConn1 -- Spatial Contact Force3/LConn1 -- Spatial Contact Force2/LConn1 -- Spatial Contact Force1/LConn1 -- Cable_1/RConn1
  Spatial Contact Force2/RConn1 -- Spatial Contact Force17/RConn1 -- Conn6/RConn1
  Spatial Contact Force5/RConn1 -- Spatial Contact Force14/RConn1 -- Conn12/RConn1
  Spatial Contact Force4/RConn1 -- Spatial Contact Force15/RConn1 -- Conn10/RConn1
  Spatial Contact Force3/RConn1 -- Spatial Contact Force16/RConn1 -- Conn8/RConn1
  Spatial Contact Force6/RConn1 -- Spatial Contact Force13/RConn1 -- Conn14/RConn1
  Spatial Contact Force8/RConn1 -- Spatial Contact Force11/RConn1 -- Conn18/RConn1
  Spatial Contact Force7/RConn1 -- Spatial Contact Force12/RConn1 -- Conn16/RConn1
  Spatial Contact Force9/RConn1 -- Spatial Contact Force10/RConn1 -- Conn20/RConn1
  Spatial Contact Force16/LConn1 -- Spatial Contact Force19/LConn1 -- Spatial Contact Force18/LConn1 -- Spatial Contact Force17/LConn1 -- Spatial Contact Force12/LConn1 -- Spatial Contact Force10/LConn1 -- Cable_3/RConn1 -- Spatial Contact Force11/LConn1 -- Spatial Contact Force13/LConn1 -- Spatial Contact Force14/LConn1 -- Spatial Contact Force15/LConn1

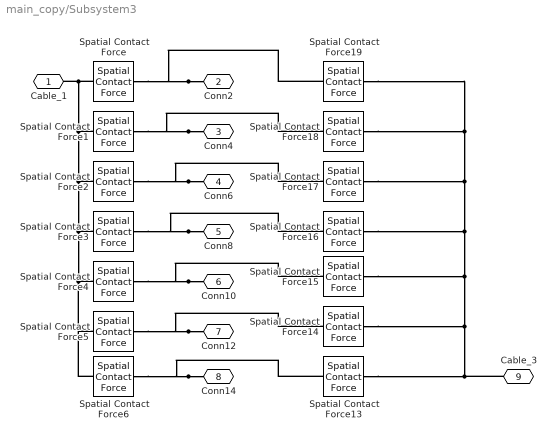
== system main_copy/Subsystem3 ==
  Spatial Contact Force{,1..6,13..19} (14 alike) : sm_lib/Forces and Torques/Spatial Contact Force  SenseContactBaseRotation=off  SenseContactBaseTranslation=off  CoefficientOfDynamicFriction=0.3  CoefficientOfStaticFriction=0.5  NormalDamping=1e3  NormalDampingUnits=N/(m/s)  SenseContactSignal=off  NormalStiffness=1e6  NormalStiffnessUnits=N/m  FrictionalCriticalVelocity=1e-3  FrictionalCriticalVelocityUnits=m/s  ZeroCrossDetectContactStartAndEnd=off  SenseContactFollowerRotation=off  SenseContactFollowerTranslation=off  FrictionType=SmoothStickSlip  SenseFrictionalForceMagnitude=off  SenseNormalForceMagnitude=off  NormalForceType=SmoothSpringDamper  SenseNormalVelocity=off  SensePenetrationDepth=off  SenseSeparationDistance=off  SenseTangentialVelocity=off  NormalTransitionRegionWidth=1e-4  NormalTransitionRegionWidthUnits=m
  Cable_1 : PMIOPort  Side=Left
  Conn2 : PMIOPort  Port=2  Side=Right
  Conn4 : PMIOPort  Port=3  Side=Right
  Conn6 : PMIOPort  Port=4  Side=Right
  Conn8 : PMIOPort  Port=5  Side=Right
  Conn10 : PMIOPort  Port=6  Side=Right
  Conn12 : PMIOPort  Port=7  Side=Right
  Conn14 : PMIOPort  Port=8  Side=Right
  Cable_3 : PMIOPort  Port=9  Side=Left
  connections:
  Conn2/RConn1 -- Spatial Contact Force/RConn1 -- Spatial Contact Force19/RConn1
  Conn4/RConn1 -- Spatial Contact Force1/RConn1 -- Spatial Contact Force18/RConn1
  Spatial Contact Force/LConn1 -- Cable_1/RConn1 -- Spatial Contact Force1/LConn1 -- Spatial Contact Force2/LConn1 -- Spatial Contact Force3/LConn1 -- Spatial Contact Force4/LConn1 -- Spatial Contact Force6/LConn1 -- Spatial Contact Force5/LConn1
  Conn6/RConn1 -- Spatial Contact Force2/RConn1 -- Spatial Contact Force17/RConn1
  Conn12/RConn1 -- Spatial Contact Force5/RConn1 -- Spatial Contact Force14/RConn1
  Conn10/RConn1 -- Spatial Contact Force4/RConn1 -- Spatial Contact Force15/RConn1
  Conn8/RConn1 -- Spatial Contact Force3/RConn1 -- Spatial Contact Force16/RConn1
  Conn14/RConn1 -- Spatial Contact Force6/RConn1 -- Spatial Contact Force13/RConn1
  Spatial Contact Force19/LConn1 -- Spatial Contact Force18/LConn1 -- Spatial Contact Force17/LConn1 -- Spatial Contact Force16/LConn1 -- Spatial Contact Force15/LConn1 -- Spatial Contact Force14/LConn1 -- Cable_3/RConn1 -- Spatial Contact Force13/LConn1

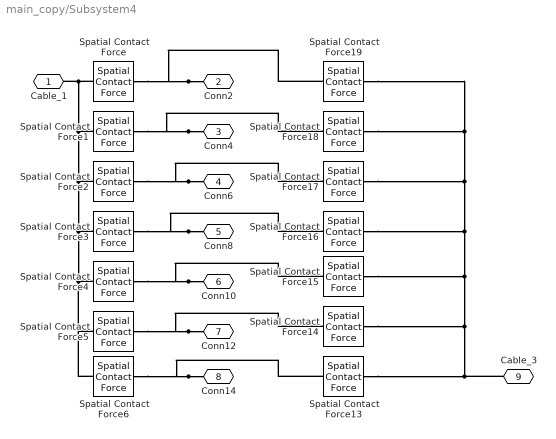
== system main_copy/Subsystem4 ==
  Spatial Contact Force{,1..6,13..19} (14 alike) : sm_lib/Forces and Torques/Spatial Contact Force  SenseContactBaseRotation=off  SenseContactBaseTranslation=off  CoefficientOfDynamicFriction=0.3  CoefficientOfStaticFriction=0.5  NormalDamping=1e3  NormalDampingUnits=N/(m/s)  SenseContactSignal=off  NormalStiffness=1e6  NormalStiffnessUnits=N/m  FrictionalCriticalVelocity=1e-3  FrictionalCriticalVelocityUnits=m/s  ZeroCrossDetectContactStartAndEnd=off  SenseContactFollowerRotation=off  SenseContactFollowerTranslation=off  FrictionType=SmoothStickSlip  SenseFrictionalForceMagnitude=off  SenseNormalForceMagnitude=off  NormalForceType=SmoothSpringDamper  SenseNormalVelocity=off  SensePenetrationDepth=off  SenseSeparationDistance=off  SenseTangentialVelocity=off  NormalTransitionRegionWidth=1e-4  NormalTransitionRegionWidthUnits=m
  Cable_1 : PMIOPort  Side=Left
  Conn2 : PMIOPort  Port=2  Side=Right
  Conn4 : PMIOPort  Port=3  Side=Right
  Conn6 : PMIOPort  Port=4  Side=Right
  Conn8 : PMIOPort  Port=5  Side=Right
  Conn10 : PMIOPort  Port=6  Side=Right
  Conn12 : PMIOPort  Port=7  Side=Right
  Conn14 : PMIOPort  Port=8  Side=Right
  Cable_3 : PMIOPort  Port=9  Side=Left
  connections:
  Conn2/RConn1 -- Spatial Contact Force/RConn1 -- Spatial Contact Force19/RConn1
  Conn4/RConn1 -- Spatial Contact Force1/RConn1 -- Spatial Contact Force18/RConn1
  Spatial Contact Force/LConn1 -- Cable_1/RConn1 -- Spatial Contact Force1/LConn1 -- Spatial Contact Force2/LConn1 -- Spatial Contact Force3/LConn1 -- Spatial Contact Force4/LConn1 -- Spatial Contact Force6/LConn1 -- Spatial Contact Force5/LConn1
  Conn6/RConn1 -- Spatial Contact Force2/RConn1 -- Spatial Contact Force17/RConn1
  Conn12/RConn1 -- Spatial Contact Force5/RConn1 -- Spatial Contact Force14/RConn1
  Conn10/RConn1 -- Spatial Contact Force4/RConn1 -- Spatial Contact Force15/RConn1
  Conn8/RConn1 -- Spatial Contact Force3/RConn1 -- Spatial Contact Force16/RConn1
  Conn14/RConn1 -- Spatial Contact Force6/RConn1 -- Spatial Contact Force13/RConn1
  Spatial Contact Force19/LConn1 -- Spatial Contact Force18/LConn1 -- Spatial Contact Force17/LConn1 -- Spatial Contact Force16/LConn1 -- Spatial Contact Force15/LConn1 -- Spatial Contact Force14/LConn1 -- Cable_3/RConn1 -- Spatial Contact Force13/LConn1

== matlab function main_copy/MATLAB Function1 ==
  data: t input; y output
function y = angle2(t)

    % Each row represents one motion:
    % [t_start, duration, y_start, y_end]

    movements = [
        1.5, 1.0,   -90,   -96;
        3.5, 2.0,  -96,   0;
        11.5, 4.0,  0,  90;
    ];

    % Initial value
    y = movements(1,3);

    % Check each motion
    for i = 1:size(movements,1)

        t_start = movements(i,1);
        duration = movements(i,2);
        y_start = movements(i,3);
        y_end = movements(i,4);

        % Before this movement
        if t <= t_start

            y = y_start;
            return

        % During this movement
        elseif t < (t_start + duration)

            % Normalized time: 0 -> 1
            tau = (t - t_start) / duration;

            % 5th-order smooth trajectory
            s = 6*tau^5 - 15*tau^4 + 10*tau^3;

            y = y_start + (y_end - y_start) * s;
            return

        % After this movement
        else

            y = y_end;

        end
    end
end

== matlab function main_copy/MATLAB Function ==
  data: t input; y output; p input
function y = fcn(t, p) 
    % ===================================================================== 
    % CONTROL PARAMETERS 
    % ===================================================================== 
    F_clamp             = -0;    % Target full clamping force (N) 
     
    % --- Initial Clamping Parameters --- 
    F_approach1         = -1;     % Gentle approach force for first clamp (N) 
    p_stiffness1        = 0.002;    % Penetration depth for full force (m) 
     
    % --- Second Clamping Parameters (Specific to final phase) --- 
    F_approach_clamp2   = -0.001;     % Gentle approach force for second clamp (N) 
    p_stiffness_clamp2  = 0.0015;   % Penetration depth for second clamp (m) 
     
    p_contact           = 0.0;      % Contact position threshold (m) 
     
    p_start             = -0.015;   % Position when clamped (m) 
    p_target            = -15e-3;     % Target release position (m) 
     
    t_release           = 0.5;      % Time to start release (s) 
    move_dur            = 0.8;      % Duration of release movement (s) 
     
    Kp                  = 150;      % Position tracking gain (N/m) 
    Kd_scale            = 0.5;      % Braking scale when overshooting 
     
    t_second_clamp      = 16.5;      % Time to re-engage clamping (s) 
    % ===================================================================== 
    p_start2 = 0.06; 
    p_target2 =0; 
     
    % 1. Initial Clamping Phase 
    if t < t_release 
        if p < p_contact 
            % Gentle approach before contact 
            y = F_approach1; 
        else 
            % Smooth force ramp upon contact based on deflection 
            contact_ratio = min(1.0, (p - p_contact) / p_stiffness1); 
            y = F_approach1 + (F_clamp - F_approach1) * contact_ratio; 
        end 
         
    % 2. S-Curve Release & Dynamic Hold Phase 
    elseif t >= t_release && t < (t_second_clamp-1.5) 
        tau = min(1.0, (t - t_release) / move_dur); 
         
        s_curve = tau^3 * (6 * tau^2 - 15 * tau + 10); 
        p_ref = p_start + (p_target - p_start) * s_curve; 
         
        err = p_ref - p; 
        p_start2=p; 
        if err >= 0 
            y = Kp * err; 
        else 
            y = Kp * err * (1 + Kd_scale * abs(err)); 
        end 
         
        if tau >= 1.0 
            if abs(p_target - p) < 0.003 
                y = y * (abs(p_target - p) / 0.003); 
            end 
        end 
         
    % 3. Second Clamping Phase (t >= t_second_clamp) 
    elseif t > (t_second_clamp-1.5)  && t <t_second_clamp 
        tau = min(1.0, (t - (t_second_clamp-1.5)) / move_dur); 
         
        s_curve = tau^3 * (6 * tau^2 - 15 * tau + 10); 
        p_ref = p_start2 + (p_target2 - p_start2) * s_curve; 
         
        err = p_ref - p; 
         
        if err >= 0 
            y = Kp * err; 
        else 
            y = Kp * err * (1 + Kd_scale * abs(err)); 
        end 
         
        if tau >= 1.0 
            if abs(p_target2 - p) < 0.003 
                y = y * (abs(p_target2 - p) / 0.003); 
            end 
        end 
    else 
        y = -500; 
    end 
end

== matlab function main_copy/MATLAB Function2 ==
  data: t input; y output

function y = angle2(t)

    % Each row represents one motion:
    % [t_start, duration, y_start, y_end]

    movements = [
      
        1.5, 1.0,   0,   -6;
        5.5, 4.0,   -6,   186;

    ];

    % Initial position
    y = movements(1,3);

    % Check each movement
    for i = 1:size(movements,1)

        t_start = movements(i,1);
        duration = movements(i,2);
        y_start = movements(i,3);
        y_end = movements(i,4);

        if t <= t_start

            % Before movement starts
            y = y_start;
            return

        elseif t < (t_start + duration)

            % During movement
            tau = (t - t_start) / duration;

            % 5th-order smooth trajectory
            s = 6*tau^5 - 15*tau^4 + 10*tau^3;

            y = y_start + (y_end - y_start) * s;
            return

        else

            % Movement completed
            y = y_end;

        end
    end
end

== matlab function main_copy/MATLAB Function4 ==
  data: t input; y output
function y = angle(t)

    % Each row represents one movement:
    % [t_start, duration, y_start, y_end]

    movements = [
        3.0, 0.5,   -90-25.5,   -90;
      
    ];

    % Default value
    y = movements(1,3);

    % Check each movement
    for i = 1:size(movements,1)

        t_start = movements(i,1);
        duration = movements(i,2);
        y_start = movements(i,3);
        y_end = movements(i,4);

        if t <= t_start
            y = y_start;
            return

        elseif t < (t_start + duration)

            % Normalized time
            tau = (t - t_start) / duration;

            % 5th-order smooth polynomial
            s = 6*tau^5 - 15*tau^4 + 10*tau^3;

            y = y_start + (y_end - y_start) * s;
            return

        else
            % Movement is complete
            y = y_end;
        end
    end
end
